simulink model "lpf"  (R2023a)
settings: Solver=VariableStepAuto  StartTime=0.0  StopTime=10.0  RelTol=1e-3
libraries: simulink x2
settings Model: Creator=andykim02  LastModifiedBy=andykim02
settings SFSimCC: SimCustomHeaderCode="#include \"LPF.h\""  SimUserSources=lpf.c

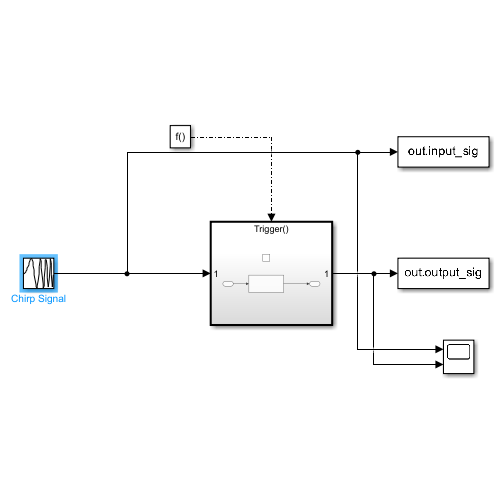
[thumbnail: Simulink's stored preview of the top-level diagram]
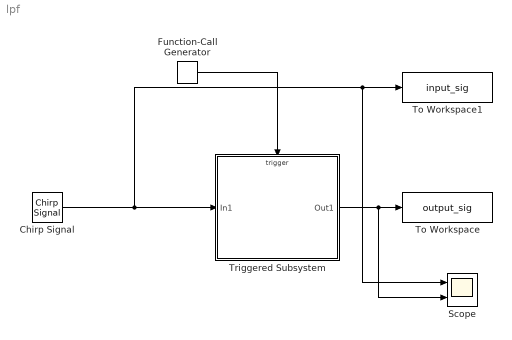
== system lpf ==
  Chirp Signal : simulink/Sources/Chirp Signal  f1=10  T=1  f2=1000
  Function-Call Generator : simulink/Ports & Subsystems/Function-Call Generator  sample_time=1e-4  numberOfIterations=1  DisallowWideOutput=off
  Scope : Scope  NumInputPorts=2
  To Workspace : ToWorkspace  VariableName=output_sig  SampleTime=-1
  To Workspace1 : ToWorkspace  VariableName=input_sig  SampleTime=-1
  Triggered Subsystem : Subsystem  TreatAsAtomicUnit=on
  wires:
  Function-Call Generator/1 -> Triggered Subsystem/Trigger
  Triggered Subsystem/1(Out1) -> Scope/2, To Workspace/1
  Chirp Signal/1 -> Scope/1, To Workspace1/1, Triggered Subsystem/1(In1)

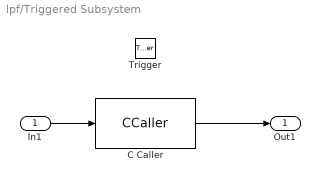
== system lpf/Triggered Subsystem ==
  In1 : Inport
  Trigger : TriggerPort  TriggerType=function-call  VariantControl=(inherit)
  C Caller : CCaller  FunctionName=LPF_Update  PortSpecificationStruct="%)30     .    R ,   8    (     @         %    \"     (    !     0         %  0 \"0    $    _    07)G3F%M90  4&]R=$YA;64 4V-O<&4     26YD97@     5'EP90      4VEZ90      27-';&]B86P   X    P    !@    @    $          4    (     0    ,    !         !   P!O=70 #@   #     &    \"     0         !0    @    !     P    $         $  # &]U=  .    .     8    (    !          %    \"     $    &     0         0    !@   $]U='!U=   #@   #@    &    \"     8         !0    @    !     0    $         \"0    @               X    X    !@    @    $          4    (     0    8    !         !     &    9&]U8FQE   .    ,     8    (    !          %    \"     $    !     0         0  $ ,0    X    P    !@    @    ) @        4    (     0    $    !          (  0      #@   #@    &    \"     0         !0    @    !    !0    $         $     4   !I;G!U=     X    X    !@    @    $          4    (     0    4    !         !     %    :6YP=70    .    .     8    (    !          %    \"     $    %     0         0    !0   $EN<'5T    #@   #@    &    \"     8         !0    @    !     0    $         \"0    @               X    X    !@    @    $          4    (     0    8    !         !     &    9&]U8FQE   .    ,     8    (    !          %    \"     $    !     0         0  $ ,0    X    P    !@    @    ) @        4    (     0    $    !          (  0"
  Out1 : Outport
  wires:
  In1/1 -> C Caller/1
  C Caller/1 -> Out1/1
